simulink model "TMW_demo_SimpleJavaCall"  (Simulink 7.9)
settings: Solver=FixedStepDiscrete  StartTime=0.0  StopTime=1  RelTol=1e-3
undefined symbols (not defined in the file or in its folder): XData, YData
libraries: realtime_pacer_lib x1
settings Model: Creator=The MathWorks Inc.  LastModifiedBy=tfsteven  ExtModeTrigMode=oneshot  ExtModeArmWhenConnect=off  ExtModeAutoUpdateStatusClock=off
settings DataIOCC: LimitDataPoints=off
settings OptimizationCC: BooleanDataType=off  InlineInvariantSignals=on  InitFltsAndDblsToZero=on
settings DebuggingCC: SaveWithParameterizedLinksMsg=none  SignalResolutionControl=TryResolveAllWithWarning  SolverPrmCheckMsg=none  MultiTaskDSMMsg=warning  MultiTaskCondExecSysMsg=none  FcnCallInpInsideContextMsg=Use local settings
settings HardwareCC: TargetUnknown=on
settings RTWCC: IncludeERTFirstTime=on
settings GRTTargetCC: TargetFcnLib=ansi_tfl_tmw.mat  CombineOutputUpdateFcns=off  GRTInterface=on

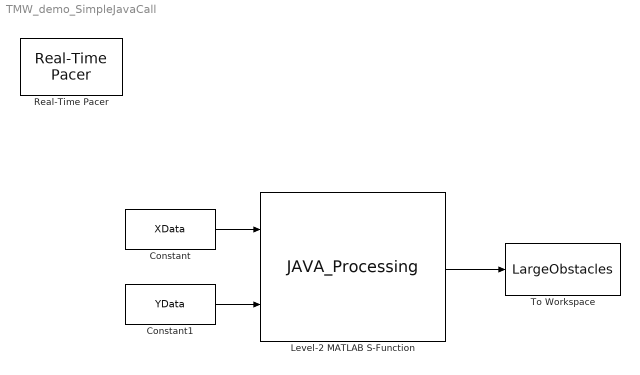
== system TMW_demo_SimpleJavaCall ==
  Constant : Constant  Value=XData  VectorParams1D=off
  Constant1 : Constant  Value=YData  VectorParams1D=off
  Level-2 MATLAB S-Function : M-S-Function  FunctionName=JAVA_Processing  Parameters=1000,50,725
  Real-Time Pacer : realtime_pacer_lib/Real-Time Pacer  simTimePerRealTime=1
  To Workspace : ToWorkspace  VariableName=LargeObstacles  SampleTime=-1
  wires:
  Level-2 MATLAB S-Function/1 -> To Workspace/1
  Constant/1 -> Level-2 MATLAB S-Function/1
  Constant1/1 -> Level-2 MATLAB S-Function/2
